simulink model "s_invert"  (Simulink 4.00)
settings: Solver=ode5  SolverMode=SingleTasking  StartTime=0.0  StopTime=60e-6  FixedStep=1e-7  MaxStep=1e-7  RelTol=1e-3  AbsTol=1e-6
libraries: simulink3 x1
settings Model: LastModifiedBy=Administrator  SaveTime=off  SaveOutput=off  LimitDataPoints=off  BlockReductionOpt=off

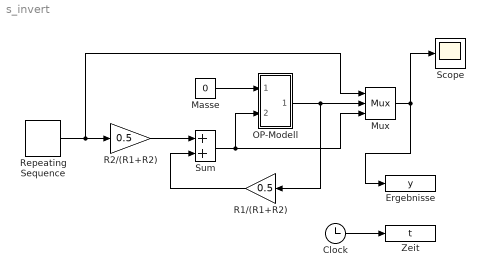
== system s_invert ==
  Clock : Clock
      settings: DisplayTime=off  Decimation=10
  Ergebnisse : ToWorkspace  VariableName=y  SampleTime=0  SaveFormat=Array
      settings: MaxDataPoints=1000
  Masse : Constant  Value=0
  Mux : Mux  Inputs=3
      settings: DisplayOption=none
  OP-Modell : Subsystem
      settings: RTWFcnNameOpts=Auto  RTWFileNameOpts=Auto
  R1/(R1+R2) : Gain  Orientation=left  Gain=0.5  Multiplication=Element-wise(K.*u)  SaturateOnIntegerOverflow=on
  R2/(R1+R2) : Gain  Gain=0.5  Multiplication=Element-wise(K.*u)  SaturateOnIntegerOverflow=on
  Repeating Sequence : simulink3/Sources/Repeating Sequence  rep_seq_t=[0, 5e-6, 10e-6, 15e-6, 20e-6]  rep_seq_y=[0 4 0 -4 0]
  Scope : Scope
      settings: TickLabels=on  TimeRange=6e-005  YMin=-1  YMax=1  SaveToWorkspace=off  SaveName=ScopeData  DataFormat=Array  LimitDataPoints=on  MaxDataPoints=5000
  Sum : Sum  Inputs=++  SaturateOnIntegerOverflow=on
  Zeit : ToWorkspace  VariableName=t  SampleTime=0  SaveFormat=Array
      settings: MaxDataPoints=1000
  wires:
  Mux/1 -> Scope/1, Ergebnisse/1
  Clock/1 -> Zeit/1
  Sum/1 -> Mux/3, OP-Modell/2(in_2)
  OP-Modell/1(out_1) -> Mux/2, R1/(R1+R2)/1
  Repeating Sequence/1 -> Mux/1, R2/(R1+R2)/1
  R2/(R1+R2)/1 -> Sum/1
  R1/(R1+R2)/1 -> Sum/2
  Masse/1 -> OP-Modell/1(in_1)

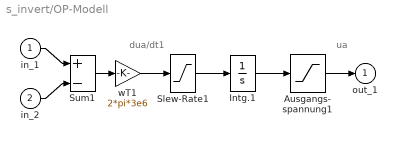
== system s_invert/OP-Modell ==
  note: ua
  note: dua/dt1
  in_1 : Inport  Port=1
  in_2 : Inport  Port=2
  " wT1" : Gain  Gain=2*pi*3e6  Multiplication=Element-wise(K.*u)  SaturateOnIntegerOverflow=on
  Ausgangs- spannung1 : Saturate  UpperLimit=10  LowerLimit=-10  LinearizeAsGain=on
  Intg.1 : Integrator  ExternalReset=none  InitialConditionSource=internal  InitialCondition=0  LimitOutput=off  UpperSaturationLimit=inf  LowerSaturationLimit=-inf  ShowSaturationPort=off  ShowStatePort=off  AbsoluteTolerance=auto
  Slew-Rate1 : Saturate  UpperLimit=1e6  LowerLimit=-1e6  LinearizeAsGain=on
  Sum1 : Sum  Inputs=+-  SaturateOnIntegerOverflow=on
  out_1 : Outport  Port=1
  wires:
  Intg.1/1 -> Ausgangs- spannung1/1
  Slew-Rate1/1 -> Intg.1/1
  " wT1"/1 -> Slew-Rate1/1
  Sum1/1 -> " wT1"/1
  in_1/1 -> Sum1/1
  Ausgangs- spannung1/1 -> out_1/1
  in_2/1 -> Sum1/2
